simulink model "FIR_fda_pipe"  (R2015b)
settings: Solver=FixedStepDiscrete  SolverMode=SingleTasking  StartTime=0.0  StopTime=10000/1e6  RelTol=1e-3
libraries: simulink x1
settings Model: Creator=at-mt  LastModifiedBy=amatsumo
settings DataIOCC: SaveFormat=Array  SignalLoggingSaveFormat=ModelDataLogs  SaveOutput=off  SignalLogging=off  SaveTime=off
settings OptimizationCC: BlockReduction=off  ConditionallyExecuteInputs=off  DefaultParameterBehavior=Inlined  ExpressionDepthLimit=2147483647
settings DebuggingCC: AlgebraicLoopMsg=error  UnderspecifiedInitializationDetection=Classic  MergeDetectMultiDrivingBlocksExec=none  SolverPrmCheckMsg=warning  InheritedTsInSrcMsg=none  SingleTaskRateTransMsg=error  FcnCallInpInsideContextMsg=UseLocalSettings  StateNameClashWarn=warning
settings HardwareCC: ProdBitPerPointer=32  ProdLargestAtomicFloat=None  ProdIntDivRoundTo=Undefined  ProdEndianess=Unspecified  ProdWordSize=32  ProdHWDeviceType=ASIC/FPGA->ASIC/FPGA  ProdEqTarget=off
settings GRTTargetCC: GeneratePreprocessorConditionals=Disable all  CombineOutputUpdateFcns=off  GRTInterface=on
settings ConfigComp: CovModelRefEnable=Off  CovSFcnEnable=off

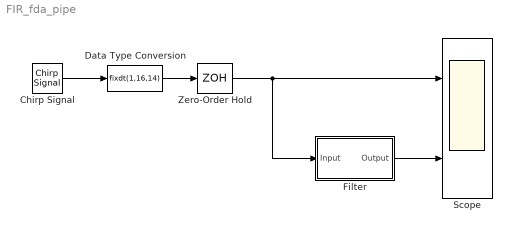
== system FIR_fda_pipe ==
  Chirp Signal : simulink/Sources/Chirp Signal  f1=10e3  T=10000/1e6  f2=500e3
  Data Type Conversion : DataTypeConversion  OutDataTypeStr=fixdt(1,16,14)  RndMeth=Nearest
  Filter : Subsystem  Tag=FilterWizardSubSystem
      settings: ErrorFcn=dspFilterRealizedInBasicElemsAlgLoopErrFcnCallback
  Scope : Scope  NumInputPorts=2
  Zero-Order Hold : ZeroOrderHold  SampleTime=1/1e6
  wires:
  Filter/1(Output) -> Scope/2
  Zero-Order Hold/1 -> Filter/1(Input), Scope/1
  Chirp Signal/1 -> Data Type Conversion/1
  Data Type Conversion/1 -> Zero-Order Hold/1

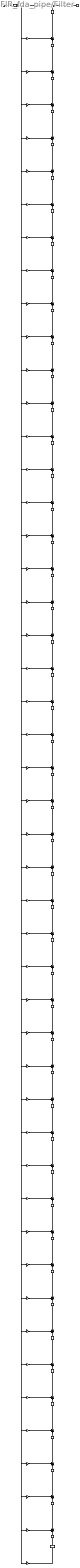
== system FIR_fda_pipe/Filter ==
  Input : Inport
  BodyRDelay{2..48} (47 alike) : Delay  DelayLength=1  InitialCondition=0  InputProcessing=Columns as channels (frame based)
  BodyRSum{2..47} (46 alike) : Sum  Inputs=++|  AccumDataTypeStr=fixdt(1,33,30)  OutDataTypeStr=fixdt(1,33,31)
  ConvertIn : DataTypeConversion  OutDataTypeStr=fixdt(1,16,14)  RndMeth=Nearest  SaturateOnIntegerOverflow=on
  ConvertOut : DataTypeConversion  OutDataTypeStr=fixdt(1,16,14)
  ConvertState48 : DataTypeConversion  OutDataTypeStr=fixdt(1,33,31)
  HeadSumR1 : Sum  Inputs=|++  AccumDataTypeStr=fixdt(1,33,30)  OutDataTypeStr=fixdt(1,33,31)
  b(1) : Gain  Gain=-0.0015246255854119901  ParamDataTypeStr=fixdt(1,16,16)  OutDataTypeStr=fixdt(1,31,31)
  b(10) : Gain  Gain=0.011598387637803855  ParamDataTypeStr=fixdt(1,16,16)  OutDataTypeStr=fixdt(1,31,31)
  b(11) : Gain  Gain=-0.0031016131441193155  ParamDataTypeStr=fixdt(1,16,16)  OutDataTypeStr=fixdt(1,31,31)
  b(12) : Gain  Gain=-0.01699091246940064  ParamDataTypeStr=fixdt(1,16,16)  OutDataTypeStr=fixdt(1,31,31)
  b(13) : Gain  Gain=-0.003469463473475945  ParamDataTypeStr=fixdt(1,16,16)  OutDataTypeStr=fixdt(1,31,31)
  b(14) : Gain  Gain=0.021317820921314172  ParamDataTypeStr=fixdt(1,16,16)  OutDataTypeStr=fixdt(1,31,31)
  b(15) : Gain  Gain=0.014205217299065596  ParamDataTypeStr=fixdt(1,16,16)  OutDataTypeStr=fixdt(1,31,31)
  b(16) : Gain  Gain=-0.022739848971926518  ParamDataTypeStr=fixdt(1,16,16)  OutDataTypeStr=fixdt(1,31,31)
  b(17) : Gain  Gain=-0.029832087938286563  ParamDataTypeStr=fixdt(1,16,16)  OutDataTypeStr=fixdt(1,31,31)
  b(18) : Gain  Gain=0.018638954412635484  ParamDataTypeStr=fixdt(1,16,16)  OutDataTypeStr=fixdt(1,31,31)
  b(19) : Gain  Gain=0.052011508906959603  ParamDataTypeStr=fixdt(1,16,16)  OutDataTypeStr=fixdt(1,31,31)
  b(2) : Gain  Gain=-0.0056040694699944459  ParamDataTypeStr=fixdt(1,16,16)  OutDataTypeStr=fixdt(1,31,31)
  b(20) : Gain  Gain=-0.0039935685035125054  ParamDataTypeStr=fixdt(1,16,16)  OutDataTypeStr=fixdt(1,31,31)
  b(21) : Gain  Gain=-0.087482017884039157  ParamDataTypeStr=fixdt(1,16,16)  OutDataTypeStr=fixdt(1,31,31)
  b(22) : Gain  Gain=-0.039025075223248162  ParamDataTypeStr=fixdt(1,16,16)  OutDataTypeStr=fixdt(1,31,31)
  b(23) : Gain  Gain=0.18476516322082137  ParamDataTypeStr=fixdt(1,16,16)  OutDataTypeStr=fixdt(1,31,31)
  b(24) : Gain  Gain=0.40580167040079751  ParamDataTypeStr=fixdt(1,16,16)  OutDataTypeStr=fixdt(1,31,31)
  b(25) : Gain  Gain=0.40580167040079751  ParamDataTypeStr=fixdt(1,16,16)  OutDataTypeStr=fixdt(1,31,31)
  b(26) : Gain  Gain=0.18476516322082137  ParamDataTypeStr=fixdt(1,16,16)  OutDataTypeStr=fixdt(1,31,31)
  b(27) : Gain  Gain=-0.039025075223248162  ParamDataTypeStr=fixdt(1,16,16)  OutDataTypeStr=fixdt(1,31,31)
  b(28) : Gain  Gain=-0.087482017884039157  ParamDataTypeStr=fixdt(1,16,16)  OutDataTypeStr=fixdt(1,31,31)
  b(29) : Gain  Gain=-0.0039935685035125054  ParamDataTypeStr=fixdt(1,16,16)  OutDataTypeStr=fixdt(1,31,31)
  b(3) : Gain  Gain=-0.0058450039381682788  ParamDataTypeStr=fixdt(1,16,16)  OutDataTypeStr=fixdt(1,31,31)
  b(30) : Gain  Gain=0.052011508906959603  ParamDataTypeStr=fixdt(1,16,16)  OutDataTypeStr=fixdt(1,31,31)
  b(31) : Gain  Gain=0.018638954412635484  ParamDataTypeStr=fixdt(1,16,16)  OutDataTypeStr=fixdt(1,31,31)
  b(32) : Gain  Gain=-0.029832087938286563  ParamDataTypeStr=fixdt(1,16,16)  OutDataTypeStr=fixdt(1,31,31)
  b(33) : Gain  Gain=-0.022739848971926518  ParamDataTypeStr=fixdt(1,16,16)  OutDataTypeStr=fixdt(1,31,31)
  b(34) : Gain  Gain=0.014205217299065596  ParamDataTypeStr=fixdt(1,16,16)  OutDataTypeStr=fixdt(1,31,31)
  b(35) : Gain  Gain=0.021317820921314172  ParamDataTypeStr=fixdt(1,16,16)  OutDataTypeStr=fixdt(1,31,31)
  b(36) : Gain  Gain=-0.003469463473475945  ParamDataTypeStr=fixdt(1,16,16)  OutDataTypeStr=fixdt(1,31,31)
  b(37) : Gain  Gain=-0.01699091246940064  ParamDataTypeStr=fixdt(1,16,16)  OutDataTypeStr=fixdt(1,31,31)
  b(38) : Gain  Gain=-0.0031016131441193155  ParamDataTypeStr=fixdt(1,16,16)  OutDataTypeStr=fixdt(1,31,31)
  b(39) : Gain  Gain=0.011598387637803855  ParamDataTypeStr=fixdt(1,16,16)  OutDataTypeStr=fixdt(1,31,31)
  b(4) : Gain  Gain=-6.2680724829390806e-05  ParamDataTypeStr=fixdt(1,16,16)  OutDataTypeStr=fixdt(1,31,31)
  b(40) : Gain  Gain=0.0062328738643254028  ParamDataTypeStr=fixdt(1,16,16)  OutDataTypeStr=fixdt(1,31,31)
  b(41) : Gain  Gain=-0.0064654391449295058  ParamDataTypeStr=fixdt(1,16,16)  OutDataTypeStr=fixdt(1,31,31)
  b(42) : Gain  Gain=-0.0067957421209925116  ParamDataTypeStr=fixdt(1,16,16)  OutDataTypeStr=fixdt(1,31,31)
  b(43) : Gain  Gain=0.0024746345997378864  ParamDataTypeStr=fixdt(1,16,16)  OutDataTypeStr=fixdt(1,31,31)
  b(44) : Gain  Gain=0.0059777568571996731  ParamDataTypeStr=fixdt(1,16,16)  OutDataTypeStr=fixdt(1,31,31)
  b(45) : Gain  Gain=-6.2680724829390806e-05  ParamDataTypeStr=fixdt(1,16,16)  OutDataTypeStr=fixdt(1,31,31)
  b(46) : Gain  Gain=-0.0058450039381682788  ParamDataTypeStr=fixdt(1,16,16)  OutDataTypeStr=fixdt(1,31,31)
  b(47) : Gain  Gain=-0.0056040694699944459  ParamDataTypeStr=fixdt(1,16,16)  OutDataTypeStr=fixdt(1,31,31)
  b(48) : Gain  Gain=-0.0015246255854119901  ParamDataTypeStr=fixdt(1,16,16)  OutDataTypeStr=fixdt(1,31,31)
  b(5) : Gain  Gain=0.0059777568571996731  ParamDataTypeStr=fixdt(1,16,16)  OutDataTypeStr=fixdt(1,31,31)
  b(6) : Gain  Gain=0.0024746345997378864  ParamDataTypeStr=fixdt(1,16,16)  OutDataTypeStr=fixdt(1,31,31)
  b(7) : Gain  Gain=-0.0067957421209925116  ParamDataTypeStr=fixdt(1,16,16)  OutDataTypeStr=fixdt(1,31,31)
  b(8) : Gain  Gain=-0.0064654391449295058  ParamDataTypeStr=fixdt(1,16,16)  OutDataTypeStr=fixdt(1,31,31)
  b(9) : Gain  Gain=0.0062328738643254028  ParamDataTypeStr=fixdt(1,16,16)  OutDataTypeStr=fixdt(1,31,31)
  Output : Outport
  wires:
  Input/1 -> ConvertIn/1
  b(1)/1 -> HeadSumR1/1
  HeadSumR1/1 -> ConvertOut/1
  ConvertIn/1 -> b(1)/1, b(2)/1, b(3)/1, b(4)/1, b(5)/1, b(6)/1, b(7)/1, b(8)/1, b(9)/1, b(10)/1, b(11)/1, b(12)/1, b(13)/1, b(14)/1, b(15)/1, b(16)/1, b(17)/1, b(18)/1, b(19)/1, b(20)/1, b(21)/1, b(22)/1, b(23)/1, b(24)/1, b(25)/1, b(26)/1, b(27)/1, b(28)/1, b(29)/1, b(30)/1, b(31)/1, b(32)/1, b(33)/1, b(34)/1, b(35)/1, b(36)/1, b(37)/1, b(38)/1, b(39)/1, b(40)/1, b(41)/1, b(42)/1, b(43)/1, b(44)/1, b(45)/1, b(46)/1, b(47)/1, b(48)/1
  ConvertOut/1 -> Output/1
  b(2)/1 -> BodyRSum2/1
  BodyRSum2/1 -> BodyRDelay2/1
  BodyRDelay2/1 -> HeadSumR1/2
  b(3)/1 -> BodyRSum3/1
  BodyRSum3/1 -> BodyRDelay3/1
  BodyRDelay3/1 -> BodyRSum2/2
  b(4)/1 -> BodyRSum4/1
  BodyRSum4/1 -> BodyRDelay4/1
  BodyRDelay4/1 -> BodyRSum3/2
  b(5)/1 -> BodyRSum5/1
  BodyRSum5/1 -> BodyRDelay5/1
  BodyRDelay5/1 -> BodyRSum4/2
  b(6)/1 -> BodyRSum6/1
  BodyRSum6/1 -> BodyRDelay6/1
  BodyRDelay6/1 -> BodyRSum5/2
  b(7)/1 -> BodyRSum7/1
  BodyRSum7/1 -> BodyRDelay7/1
  BodyRDelay7/1 -> BodyRSum6/2
  b(8)/1 -> BodyRSum8/1
  BodyRSum8/1 -> BodyRDelay8/1
  BodyRDelay8/1 -> BodyRSum7/2
  b(9)/1 -> BodyRSum9/1
  BodyRSum9/1 -> BodyRDelay9/1
  BodyRDelay9/1 -> BodyRSum8/2
  b(10)/1 -> BodyRSum10/1
  BodyRSum10/1 -> BodyRDelay10/1
  BodyRDelay10/1 -> BodyRSum9/2
  b(11)/1 -> BodyRSum11/1
  BodyRSum11/1 -> BodyRDelay11/1
  BodyRDelay11/1 -> BodyRSum10/2
  b(12)/1 -> BodyRSum12/1
  BodyRSum12/1 -> BodyRDelay12/1
  BodyRDelay12/1 -> BodyRSum11/2
  b(13)/1 -> BodyRSum13/1
  BodyRSum13/1 -> BodyRDelay13/1
  BodyRDelay13/1 -> BodyRSum12/2
  b(14)/1 -> BodyRSum14/1
  BodyRSum14/1 -> BodyRDelay14/1
  BodyRDelay14/1 -> BodyRSum13/2
  b(15)/1 -> BodyRSum15/1
  BodyRSum15/1 -> BodyRDelay15/1
  BodyRDelay15/1 -> BodyRSum14/2
  b(16)/1 -> BodyRSum16/1
  BodyRSum16/1 -> BodyRDelay16/1
  BodyRDelay16/1 -> BodyRSum15/2
  b(17)/1 -> BodyRSum17/1
  BodyRSum17/1 -> BodyRDelay17/1
  BodyRDelay17/1 -> BodyRSum16/2
  b(18)/1 -> BodyRSum18/1
  BodyRSum18/1 -> BodyRDelay18/1
  BodyRDelay18/1 -> BodyRSum17/2
  b(19)/1 -> BodyRSum19/1
  BodyRSum19/1 -> BodyRDelay19/1
  BodyRDelay19/1 -> BodyRSum18/2
  b(20)/1 -> BodyRSum20/1
  BodyRSum20/1 -> BodyRDelay20/1
  BodyRDelay20/1 -> BodyRSum19/2
  b(21)/1 -> BodyRSum21/1
  BodyRSum21/1 -> BodyRDelay21/1
  BodyRDelay21/1 -> BodyRSum20/2
  b(22)/1 -> BodyRSum22/1
  BodyRSum22/1 -> BodyRDelay22/1
  BodyRDelay22/1 -> BodyRSum21/2
  b(23)/1 -> BodyRSum23/1
  BodyRSum23/1 -> BodyRDelay23/1
  BodyRDelay23/1 -> BodyRSum22/2
  b(24)/1 -> BodyRSum24/1
  BodyRSum24/1 -> BodyRDelay24/1
  BodyRDelay24/1 -> BodyRSum23/2
  b(25)/1 -> BodyRSum25/1
  BodyRSum25/1 -> BodyRDelay25/1
  BodyRDelay25/1 -> BodyRSum24/2
  b(26)/1 -> BodyRSum26/1
  BodyRSum26/1 -> BodyRDelay26/1
  BodyRDelay26/1 -> BodyRSum25/2
  b(27)/1 -> BodyRSum27/1
  BodyRSum27/1 -> BodyRDelay27/1
  BodyRDelay27/1 -> BodyRSum26/2
  b(28)/1 -> BodyRSum28/1
  BodyRSum28/1 -> BodyRDelay28/1
  BodyRDelay28/1 -> BodyRSum27/2
  b(29)/1 -> BodyRSum29/1
  BodyRSum29/1 -> BodyRDelay29/1
  BodyRDelay29/1 -> BodyRSum28/2
  b(30)/1 -> BodyRSum30/1
  BodyRSum30/1 -> BodyRDelay30/1
  BodyRDelay30/1 -> BodyRSum29/2
  b(31)/1 -> BodyRSum31/1
  BodyRSum31/1 -> BodyRDelay31/1
  BodyRDelay31/1 -> BodyRSum30/2
  b(32)/1 -> BodyRSum32/1
  BodyRSum32/1 -> BodyRDelay32/1
  BodyRDelay32/1 -> BodyRSum31/2
  b(33)/1 -> BodyRSum33/1
  BodyRSum33/1 -> BodyRDelay33/1
  BodyRDelay33/1 -> BodyRSum32/2
  b(34)/1 -> BodyRSum34/1
  BodyRSum34/1 -> BodyRDelay34/1
  BodyRDelay34/1 -> BodyRSum33/2
  b(35)/1 -> BodyRSum35/1
  BodyRSum35/1 -> BodyRDelay35/1
  BodyRDelay35/1 -> BodyRSum34/2
  b(36)/1 -> BodyRSum36/1
  BodyRSum36/1 -> BodyRDelay36/1
  BodyRDelay36/1 -> BodyRSum35/2
  b(37)/1 -> BodyRSum37/1
  BodyRSum37/1 -> BodyRDelay37/1
  BodyRDelay37/1 -> BodyRSum36/2
  b(38)/1 -> BodyRSum38/1
  BodyRSum38/1 -> BodyRDelay38/1
  BodyRDelay38/1 -> BodyRSum37/2
  b(39)/1 -> BodyRSum39/1
  BodyRSum39/1 -> BodyRDelay39/1
  BodyRDelay39/1 -> BodyRSum38/2
  b(40)/1 -> BodyRSum40/1
  BodyRSum40/1 -> BodyRDelay40/1
  BodyRDelay40/1 -> BodyRSum39/2
  b(41)/1 -> BodyRSum41/1
  BodyRSum41/1 -> BodyRDelay41/1
  BodyRDelay41/1 -> BodyRSum40/2
  b(42)/1 -> BodyRSum42/1
  BodyRSum42/1 -> BodyRDelay42/1
  BodyRDelay42/1 -> BodyRSum41/2
  b(43)/1 -> BodyRSum43/1
  BodyRSum43/1 -> BodyRDelay43/1
  BodyRDelay43/1 -> BodyRSum42/2
  b(44)/1 -> BodyRSum44/1
  BodyRSum44/1 -> BodyRDelay44/1
  BodyRDelay44/1 -> BodyRSum43/2
  b(45)/1 -> BodyRSum45/1
  BodyRSum45/1 -> BodyRDelay45/1
  BodyRDelay45/1 -> BodyRSum44/2
  b(46)/1 -> BodyRSum46/1
  BodyRSum46/1 -> BodyRDelay46/1
  BodyRDelay46/1 -> BodyRSum45/2
  b(47)/1 -> BodyRSum47/1
  BodyRSum47/1 -> BodyRDelay47/1
  BodyRDelay47/1 -> BodyRSum46/2
  b(48)/1 -> ConvertState48/1
  BodyRDelay48/1 -> BodyRSum47/2
  ConvertState48/1 -> BodyRDelay48/1
